simulink model "Buck_boost"  (R2018a)
settings: Solver=VariableStepAuto  StartTime=0.0  StopTime=2  MaxStep=0.01  RelTol=1e-4  EnableMultiTasking=on
undefined symbols (not defined in the file): C, E, iL0, L, R, uC0
settings Model: Creator=Milosh Yokich  LastModifiedBy=Milosh Yokich
settings DataIOCC: LimitDataPoints=on  SaveOutput=off  SaveTime=off
settings OptimizationCC: ExpressionDepthLimit=2147483647  LifeSpan=1
settings DebuggingCC: UnderspecifiedInitializationDetection=Classic  MergeDetectMultiDrivingBlocksExec=none  FcnCallInpInsideContextMsg=warning  AllowSymbolicDim=off  StateNameClashWarn=warning  SFUnexpectedBacktrackingDiag=warning  SFNoUnconditionalDefaultTransitionDiag=warning  SFExecutionAtInitializationDiag=none
settings CodeAppCC: StateflowObjectComments=on
settings GRTTargetCC: TargetLangStandard=C89/C90 (ANSI)  GeneratePreprocessorConditionals=Disable all  CombineOutputUpdateFcns=off  GRTInterface=on

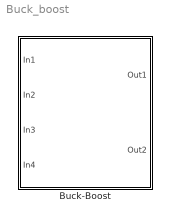
== system Buck_boost ==
  Buck-Boost : Subsystem

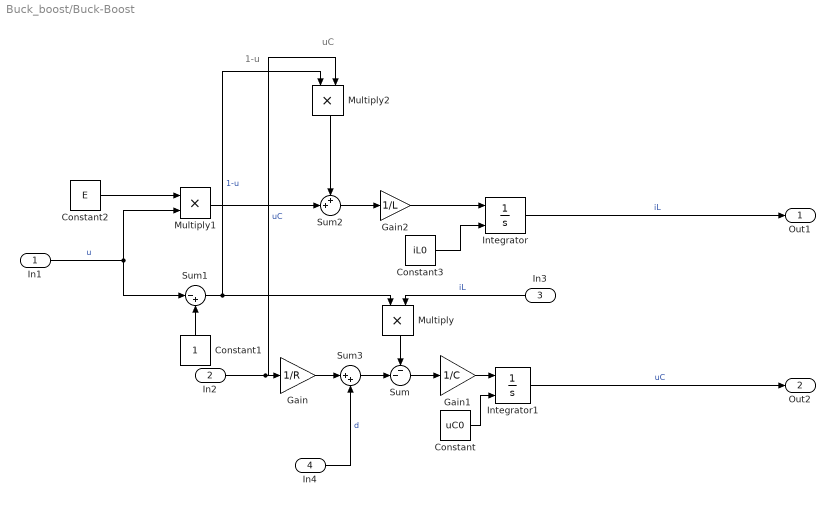
== system Buck_boost/Buck-Boost ==
  note: 1-u
  note: uC
  In1 : Inport
  In2 : Inport  Port=2
  In3 : Inport  Port=3
  In4 : Inport  Port=4
  Constant : Constant  Value=uC0
  Constant1 : Constant
  Constant2 : Constant  Value=E
  Constant3 : Constant  Value=iL0
  Gain : Gain  Gain=1/R
  Gain1 : Gain  Gain=1/C
  Gain2 : Gain  Gain=1/L
  Integrator : Integrator  InitialConditionSource=external
  Integrator1 : Integrator  InitialConditionSource=external
  Multiply : Product
  Multiply1 : Product
  Multiply2 : Product
  Sum : Sum  Inputs=--|
  Sum1 : Sum  Inputs=|-+
  Sum2 : Sum  Inputs=++|
  Sum3 : Sum  Inputs=|++
  Out1 : Outport
  Out2 : Outport  Port=2
  wires:
  Multiply2/1 -> Sum2/1
  Constant2/1 -> Multiply1/1
  Integrator1/1 -> Out2/1  "uC"
  Sum1/1 -> Multiply/1, Multiply2/1  "1-u"
  Gain2/1 -> Integrator/1
  Integrator/1 -> Out1/1  "iL"
  Gain1/1 -> Integrator1/1
  Multiply1/1 -> Sum2/2
  In1/1 -> Multiply1/2, Sum1/1  "u"
  Constant3/1 -> Integrator/2
  Multiply/1 -> Sum/1
  Constant1/1 -> Sum1/2
  Constant/1 -> Integrator1/2
  Sum/1 -> Gain1/1
  Sum2/1 -> Gain2/1
  In2/1 -> Multiply2/2, Gain/1  "uC"
  In3/1 -> Multiply/2  "iL"
  Gain/1 -> Sum3/1
  Sum3/1 -> Sum/2
  In4/1 -> Sum3/2  "d"
